simulink model "PID_houseROOMBA"  (R2024b)
settings: Solver=FixedStepAuto  StartTime=0.0  StopTime=inf  FixedStep=1/f_sim  RelTol=1e-3
model workspace (MATLAB code in the model file):
  | v_max=0.26;      % max |linear speed|
  | max_yaw=1.82;    % max |angular speed|
  | f_sim=1000;      % frequency
values from neighbouring files (symbols this model uses):
  crit_idces = -1    [Main_proj2_AstarROOMBA.m]
  path = path*res_BW-res_BW/2    [BW2GAZEBO.m]    (also in GAZEBO2BW.m = (path+res_BW/2)/res_BW; path_AstarFAST_1.mat = [-6.68726516648 -6.68556109776 -6.68385773308 -6.68215577647; path_AstarROOMBA_1.mat = [-6.7125 -6.6875 -6.6875 -6.6625 -6.6375 -6.6375 -6.6375 -6.; path_AstarROOMBA_2.mat = [4.8625 4.8375 4.8125 4.7875 4.7625 4.7375 4.7125 4.6875 4.6)
  reach_toll = 5*res    [Main_proj2_AstarFAST.m]    (also in Main_proj2_AstarROOMBA.m; Main_proj2_RRT.m = 70*mean(dist))
undefined symbols (not defined in the file or in its folder): Angular, DiscIntNeverNeededParam, Linear
libraries: robotlib x3, simulink x2, slpidlib x2
settings Model: Creator=eb  LastModifiedBy=vigno
settings OptimizationCC: DefaultParameterBehavior=Inlined  EnhancedBackFolding=on  PassReuseOutputArgsAs=Individual arguments  ZeroExternalMemoryAtStartup=off  ZeroInternalMemoryAtStartup=off  MaxStackSize=64  OptimizeBlockOrder=speed  DifferentSizesBufferReuse=on  OptimizationCustomize=off  EfficientTunableParamExpr=on
settings DebuggingCC: ParameterTunabilityLossMsg=error
settings HardwareCC: ProdBitPerPointer=32  ProdBitPerSizeT=32  ProdBitPerPtrDiffT=32  ProdLargestAtomicFloat=None  ProdIntDivRoundTo=Undefined  ProdEndianess=Unspecified  ProdWordSize=32  ProdHWDeviceType=Generic->Unspecified (assume 32-bit Generic)  UseEmbeddedCoderFeatures=off
settings SFSimCC: MATLABDynamicMemAlloc=off
settings RTWCC: Description=Embedded Coder  SystemTargetFile=ert.tlc  HardwareBoard=Robot Operating System (ROS)  TLCOptions="-aInlineSetEventsForThisBaseRateFcn=TLC_FALSE -aSuppressMultiTaskScheduler=TLC_FALSE  -aRateBasedStepFcn=0"  TemplateMakefile=ert_default_tmf  Toolchain=Catkin  TargetLang=C++
settings CodeAppCC: ForceParamTrailComments=on  IgnoreCustomStorageClasses=off  OperatorAnnotations=on  SimulinkDataObjDesc=on  SFDataObjDesc=on  InsertBlockDesc=on
settings ERTTargetCC: SupportNonInlinedSFcns=on

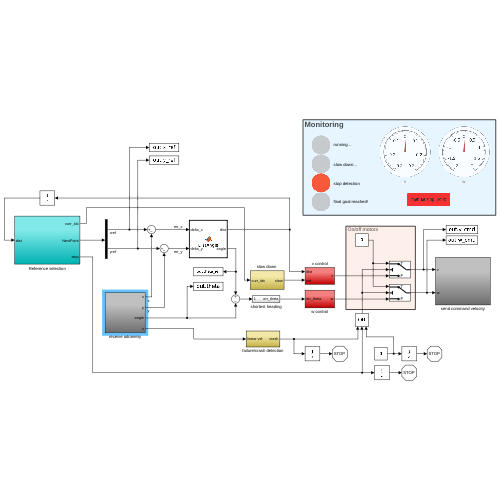
[thumbnail: Simulink's stored preview of the top-level diagram]
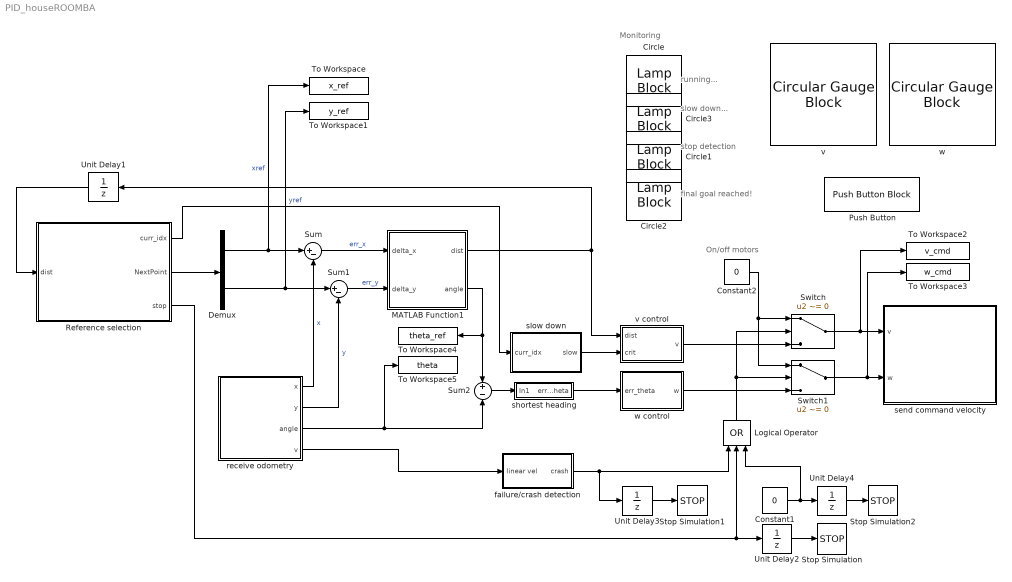
== system PID_houseROOMBA ==
  note: Monitoring
  note: running...
  note: On/off motors
  note: stop detection
  note: final goal reached!
  note: slow down...
  Circle{,1..3} (4 alike) : LampBlock  LabelPosition=Hide  Icon=Circle
  Constant1 : Constant  Value=0
  Constant2 : Constant  Value=0
  Demux : Demux  Outputs=2
  Logical Operator : Logic  Operator=OR  Inputs=3  AllPortsSameDT=off  OutDataTypeStr=boolean
  MATLAB Function1 : MATLAB Function  TreatAsAtomicUnit=on
  Push Button : PushButtonBlock  ButtonText=manual stop (hold)  OffValue=0.000000
  Reference selection : Subsystem
  Stop Simulation : Stop
  Stop Simulation1 : Stop
  Stop Simulation2 : Stop
  Sum : Sum  Inputs=|+-
  Sum1 : Sum  Inputs=|+-
  Sum2 : Sum  Inputs=+-
  Switch : Switch  Criteria=u2 ~= 0  SaturateOnIntegerOverflow=off  InputSameDT=off
  Switch1 : Switch  Criteria=u2 ~= 0  SaturateOnIntegerOverflow=off  InputSameDT=off
  To Workspace : ToWorkspace  VariableName=x_ref  SampleTime=-1
      settings: Save2DSignal=2-D array (concatenate along first dimension)
  To Workspace1 : ToWorkspace  VariableName=y_ref  SampleTime=-1
      settings: Save2DSignal=2-D array (concatenate along first dimension)
  To Workspace2 : ToWorkspace  VariableName=v_cmd  SampleTime=-1
      settings: Save2DSignal=2-D array (concatenate along first dimension)
  To Workspace3 : ToWorkspace  VariableName=w_cmd  SampleTime=-1
      settings: Save2DSignal=2-D array (concatenate along first dimension)
  To Workspace4 : ToWorkspace  VariableName=theta_ref  SampleTime=-1
      settings: Save2DSignal=2-D array (concatenate along first dimension)
  To Workspace5 : ToWorkspace  VariableName=theta  SampleTime=-1
      settings: Save2DSignal=2-D array (concatenate along first dimension)
  Unit Delay1 : UnitDelay  SampleTime=-1  HasFrameUpgradeWarning=on
  Unit Delay2 : UnitDelay  SampleTime=2  HasFrameUpgradeWarning=on
  Unit Delay3 : UnitDelay  SampleTime=0.5  HasFrameUpgradeWarning=on
  Unit Delay4 : UnitDelay  SampleTime=0.5  HasFrameUpgradeWarning=on
  failure/crash detection : Subsystem
  receive odometry : Subsystem
  send command velocity : Subsystem
  shortest heading : Subsystem
  "slow down " : Subsystem
  v : CircularGaugeBlock  LabelPosition=Hide  ScaleMin=-0.3  ScaleMax=0.3
  v control : Subsystem
  w : CircularGaugeBlock  LabelPosition=Hide  ScaleMin=-2  ScaleMax=2
  w control : Subsystem
  wires:
  Demux/1 -> Sum/1, To Workspace/1  "xref"
  Sum/1 -> MATLAB Function1/1(delta_x)  "err_x"
  Demux/2 -> Sum1/1, To Workspace1/1  "yref"
  Sum1/1 -> MATLAB Function1/2(delta_y)  "err_y"
  MATLAB Function1/2(angle) -> To Workspace4/1, Sum2/1
  MATLAB Function1/1(dist) -> v control/1(dist), Unit Delay1/1
  Sum2/1 -> shortest heading/1(In1)
  Unit Delay2/1 -> Stop Simulation/1
  Constant2/1 -> Switch1/1, Switch/1
  receive odometry/1(x) -> Sum/2  "x"
  receive odometry/2(y) -> Sum1/2  "y"
  receive odometry/3(angle) -> To Workspace5/1, Sum2/2
  Switch/1 -> To Workspace2/1, send command velocity/1(v)
  Switch1/1 -> To Workspace3/1, send command velocity/2(w)
  Reference selection/3(stop) -> Unit Delay2/1, Logical Operator/2
  Unit Delay1/1 -> Reference selection/1(dist)
  Reference selection/2(NextPoint) -> Demux/1
  receive odometry/4(v) -> failure/crash detection/1(linear vel)
  failure/crash detection/1(crash) -> Unit Delay3/1, Logical Operator/1
  Unit Delay3/1 -> Stop Simulation1/1
  Logical Operator/1 -> Switch1/2, Switch/2
  v control/1(v) -> Switch/3
  shortest heading/1(err_theta) -> w control/1(err_theta)
  "slow down "/1(slow) -> v control/2(crit)
  Reference selection/1(curr_idx) -> "slow down "/1(curr_idx)
  w control/1(w) -> Switch1/3
  Constant1/1 -> Logical Operator/3, Unit Delay4/1
  Unit Delay4/1 -> Stop Simulation2/1

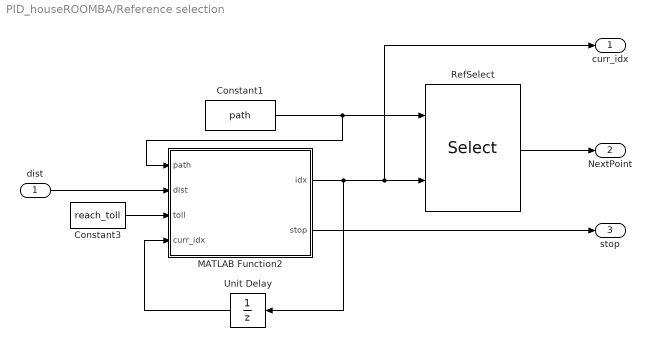
== system PID_houseROOMBA/Reference selection ==
  dist : Inport
  Constant1 : Constant  Value=path
  Constant3 : Constant  Value=reach_toll
  MATLAB Function2 : MATLAB Function  TreatAsAtomicUnit=on
  RefSelect : Selector  NumberOfDimensions=2  IndexOptions=Starting index (port),Select all  Indices=[1 3],[1:2]  OutputSizes=1,1
  Unit Delay : UnitDelay  SampleTime=-1  HasFrameUpgradeWarning=on
  curr_idx : Outport
  NextPoint : Outport  Port=2
  stop : Outport  Port=3
  wires:
  Constant3/1 -> MATLAB Function2/3(toll)
  dist/1 -> MATLAB Function2/2(dist)
  Unit Delay/1 -> MATLAB Function2/4(curr_idx)
  Constant1/1 -> MATLAB Function2/1(path), RefSelect/1
  RefSelect/1 -> NextPoint/1
  MATLAB Function2/2(stop) -> stop/1
  MATLAB Function2/1(idx) -> Unit Delay/1, curr_idx/1, RefSelect/2

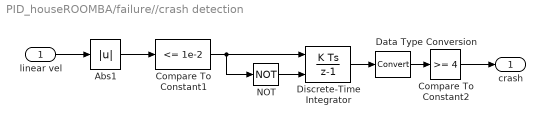
== system PID_houseROOMBA/failure//crash detection ==
  linear vel : Inport
  Abs1 : Abs  SaturateOnIntegerOverflow=off
  Compare To Constant1 : simulink/Logic and Bit Operations/Compare To Constant  relop=<=  const=1e-2  OutDataTypeStr=boolean
  Compare To Constant2 : simulink/Logic and Bit Operations/Compare To Constant  relop=>=  const=4  OutDataTypeStr=boolean
  Data Type Conversion : DataTypeConversion  SaturateOnIntegerOverflow=off  RndMeth=Floor
  Discrete-Time Integrator : DiscreteIntegrator  ExternalReset=rising  SampleTime=0.1  ICPrevOutput=DiscIntNeverNeededParam  ICPrevScaledInput=DiscIntNeverNeededParam
  NOT : Logic  Operator=NOT  IconShape=distinctive  AllPortsSameDT=off  OutDataTypeStr=boolean
  crash : Outport
  wires:
  linear vel/1 -> Abs1/1
  Abs1/1 -> Compare To Constant1/1
  Compare To Constant1/1 -> NOT/1, Discrete-Time Integrator/1
  Discrete-Time Integrator/1 -> Data Type Conversion/1
  NOT/1 -> Discrete-Time Integrator/2
  Compare To Constant2/1 -> crash/1
  Data Type Conversion/1 -> Compare To Constant2/1

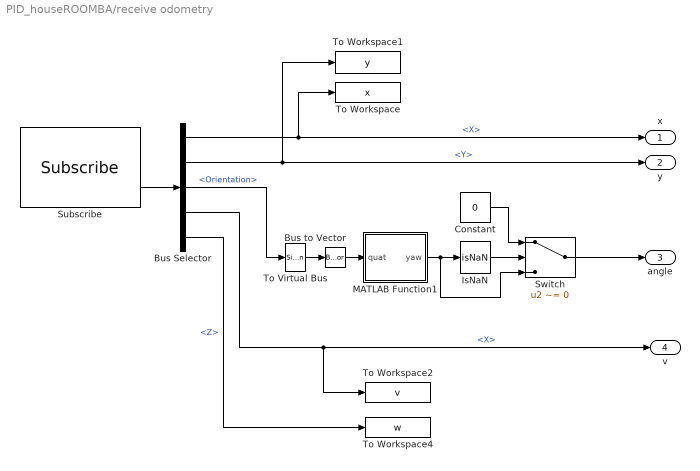
== system PID_houseROOMBA/receive odometry ==
  Bus Selector : BusSelector  OutputSignals=Pose.Pose.Position.X,Pose.Pose.Position.Y,Pose.Pose.Orientation,Twist.Twist.Linear.X,Twist.Twist.Angular.Z
  Bus to Vector : BusToVector
  Constant : Constant  Value=0
  IsNaN : RelationalOperator  Operator=isNaN  OutDataTypeStr=boolean  RndMeth=Simplest  InputSameDT=off
  MATLAB Function1 : MATLAB Function  TreatAsAtomicUnit=on
  Subscribe : robotlib/Subscribe  topicSource=Select from ROS network  topic=/odom  messageType=nav_msgs/Odometry  SampleTime=1/f_sim  legacyBusStruct=off  messageQueueLength=1
  Switch : Switch  Criteria=u2 ~= 0  SaturateOnIntegerOverflow=off  InputSameDT=off
  To Virtual Bus : SignalConversion  ConversionOutput=Virtual bus  OverrideOpt=off
  To Workspace : ToWorkspace  VariableName=x  SampleTime=-1
      settings: Save2DSignal=2-D array (concatenate along first dimension)
  To Workspace1 : ToWorkspace  VariableName=y  SampleTime=-1
      settings: Save2DSignal=2-D array (concatenate along first dimension)
  To Workspace2 : ToWorkspace  VariableName=v  SampleTime=-1
      settings: Save2DSignal=2-D array (concatenate along first dimension)
  To Workspace4 : ToWorkspace  VariableName=w  SampleTime=-1
      settings: Save2DSignal=2-D array (concatenate along first dimension)
  x : Outport
  y : Outport  Port=2
  angle : Outport  Port=3
  v : Outport  Port=4
  wires:
  Bus Selector/2 -> y/1, To Workspace1/1  "<Y>"
  Subscribe/2 -> Bus Selector/1
  Bus Selector/1 -> x/1, To Workspace/1  "<X>"
  Bus Selector/3 -> To Virtual Bus/1  "<Orientation>"
  Bus to Vector/1 -> MATLAB Function1/1(quat)
  To Virtual Bus/1 -> Bus to Vector/1
  MATLAB Function1/1(yaw) -> IsNaN/1, Switch/3
  IsNaN/1 -> Switch/2
  Constant/1 -> Switch/1
  Bus Selector/4 -> v/1, To Workspace2/1  "<X>"
  Bus Selector/5 -> To Workspace4/1  "<Z>"
  Switch/1 -> angle/1

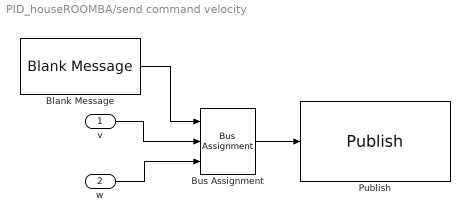
== system PID_houseROOMBA/send command velocity ==
  v : Inport
  w : Inport  Port=2
  Blank Message : robotlib/Blank Message  messageClass=Message  entityType=geometry_msgs/Twist  messageType=geometry_msgs/Twist  SampleTime=1/f_sim  legacyBusStruct=off
  Bus Assignment : BusAssignment  AssignedSignals=Linear.X,Angular.Z
  Publish : robotlib/Publish  topicSource=Select from ROS network  topic=/cmd_vel  messageType=geometry_msgs/Twist  legacyBusStruct=off  messageQueueLength=1
  wires:
  Blank Message/1 -> Bus Assignment/1
  v/1 -> Bus Assignment/2
  w/1 -> Bus Assignment/3
  Bus Assignment/1 -> Publish/1

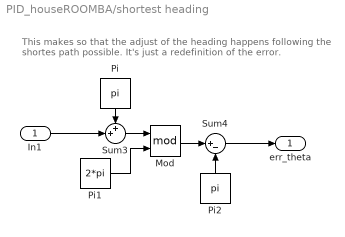
== system PID_houseROOMBA/shortest heading ==
  note: This makes so that the adjust of the heading happens following
      | the shortes path possible. It's just a redefinition of the error.
  In1 : Inport
  Mod : Math  Operator=mod
  Pi : Constant  Value=pi  OutDataTypeStr=Inherit: Inherit via back propagation
  Pi1 : Constant  Value=2*pi  OutDataTypeStr=Inherit: Inherit via back propagation
  Pi2 : Constant  Value=pi  OutDataTypeStr=Inherit: Inherit via back propagation
  Sum3 : Sum  Inputs=++|
  Sum4 : Sum  Inputs=|+-
  err_theta : Outport
  wires:
  Mod/1 -> Sum4/1
  Sum3/1 -> Mod/1
  Pi1/1 -> Mod/2
  Pi/1 -> Sum3/1
  Pi2/1 -> Sum4/2
  In1/1 -> Sum3/2
  Sum4/1 -> err_theta/1

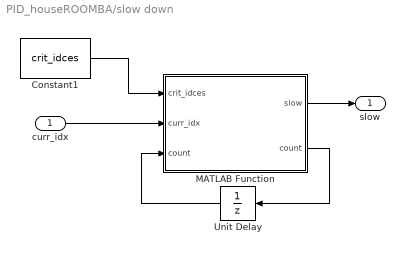
== system PID_houseROOMBA/slow down  ==
  curr_idx : Inport
  Constant1 : Constant  Value=crit_idces
  MATLAB Function : MATLAB Function  TreatAsAtomicUnit=on
  Unit Delay : UnitDelay  SampleTime=-1  HasFrameUpgradeWarning=on
  slow : Outport
  wires:
  Constant1/1 -> MATLAB Function/1(crit_idces)
  Unit Delay/1 -> MATLAB Function/3("count ")
  MATLAB Function/2(count) -> Unit Delay/1
  MATLAB Function/1(slow) -> slow/1
  curr_idx/1 -> MATLAB Function/2(curr_idx)

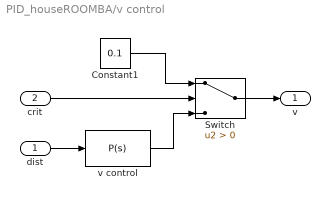
== system PID_houseROOMBA/v control ==
  dist : Inport
  crit : Inport  Port=2
  Constant1 : Constant  Value=0.1
  Switch : Switch  Criteria=u2 > Threshold  SaturateOnIntegerOverflow=off  InputSameDT=off
  v control : slpidlib/PID Controller  Controller=P  Form=Parallel  TimeDomain=Continuous-time  UseExternalTs=off  SampleTime=-1  IntegratorMethod=Forward Euler  FilterMethod=Forward Euler  ControllerParametersSource=internal  P=5  I=0.001  UseKiTs=off  D=1  UseExternalDerivativeSource=off  N=15  UseFilter=on  TunerSelectOption=Transfer Function Based (PID Tuner App)  InitialConditionSource=internal  InitialConditionForIntegrator=0  InitialConditionForFilter=0  DifferentiatorICPrevScaledInput=0  ExternalReset=none  TrackingMode=off  Kt=1  LimitOutput=on  SatLimitsSource=internal  UpperSaturationLimit=v_max  LowerSaturationLimit=-v_max  LinearizeAsGain=on  AntiWindupMode=clamping  Kb=1  LimitIntegrator=off  UpperIntegratorSaturationLimit=inf  LowerIntegratorSaturationLimit=-inf  POutMin=[]  POutMax=[]  IOutMin=[]  IOutMax=[]  DOutMin=[]  DOutMax=[]  NOutMin=[]  NOutMax=[]  SumOutMin=[]  SumOutMax=[]  SaturationOutMin=[]  SaturationOutMax=[]  PParamMin=[]  PParamMax=[]  IParamMin=[]  IParamMax=[]  DParamMin=[]  DParamMax=[]  NParamMin=[]  NParamMax=[]  KbParamMin=[]  KbParamMax=[]  KtParamMin=[]  KtParamMax=[]  KbOutMin=[]  KbOutMax=[]  KtOutMin=[]  KtOutMax=[]  IntegratorOutMin=[]  IntegratorOutMax=[]  FilterOutMin=[]  FilterOutMax=[]  SumI1OutMin=[]  SumI1OutMax=[]  SumI2OutMin=[]  SumI2OutMax=[]  SumI3OutMin=[]  SumI3OutMax=[]  SumI4OutMin=[]  SumI4OutMax=[]  SumDOutMin=[]  SumDOutMax=[]  DifferentiatorOutMin=[]  DifferentiatorOutMax=[]  FilterDiffOutCoefMin=[]  FilterDiffOutCoefMax=[]  ReciprocalOutMin=[]  ReciprocalOutMax=[]  SumDenOutMin=[]  SumDenOutMax=[]  SumNumOutMin=[]  SumNumOutMax=[]  DivideOutMin=[]  DivideOutMax=[]  UdiffTsProdOutMin=[]  UdiffTsProdOutMax=[]  NTsProdOutMin=[]  NTsProdOutMax=[]  UintegralTsProdOutMin=[]  UintegralTsProdOutMax=[]  UngainTsProdOutMin=[]  UngainTsProdOutMax=[]  ClampingZeroOutDataTypeStr=Inherit: Inherit via back propagation  ClampingZeroOutMin=[]  ClampingZeroOutMax=[]  FilterDenConstantOutDataTypeStr=Inherit: Inherit via back propagation  FilterDenConstantOutMin=[]  FilterDenConstantOutMax=[]  PCopyOutDataTypeStr=Inherit: Inherit via back propagation  PCopyOutMin=[]  PCopyOutMax=[]  NCopyOutDataTypeStr=Inherit: Inherit via back propagation  NCopyOutMin=[]  NCopyOutMax=[]  IntegratorContinuousStateAttributes=''  IntegratorStateMustResolveToSignalObject=off  IntegratorRTWStateStorageClass=Auto  FilterContinuousStateAttributes=''  FilterStateMustResolveToSignalObject=off  FilterRTWStateStorageClass=Auto  ParallelPVariant=InternalParameters  IdealPVariant=Disabled  IVariant=Disabled  DVariant=Disabled  IntegratorVariant=Disabled  SatVariant=Enabled  AWVariant=Disabled  PCopyVariant=Disabled  TRVariant=Disabled  FdbkBlocksVariant=Forward  IdealPFdbkVariant=Disabled  SatFdbkVariant=Disabled  DerivativeFilterVariant=Disabled  NVariant=Disabled  NCopyVariant=Disabled_SignalSpec  FilterICVariant=Disabled  IntegratorICVariant=Disabled  ExternalResetVariant=Disabled  TRSumVariant=Passthrough  SumFdbkVariant=Disabled  SumVariant=Passthrough_P  TsampFilterVariant=InternalTs  TsampNgainVariant=Passthrough  TsampIntegralVariant=Disabled_SignalSpec  ExternalSaturationOutDataTypeStr=Inherit: Same as second input  DerivativeSourceVariant=Disabled  PreIntVariant=InternalPreInt
  v : Outport
  wires:
  dist/1 -> v control/1
  Switch/1 -> v/1
  crit/1 -> Switch/2
  v control/1 -> Switch/3
  Constant1/1 -> Switch/1

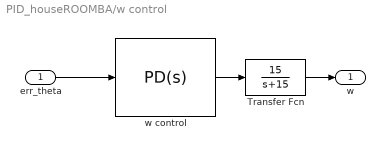
== system PID_houseROOMBA/w control ==
  err_theta : Inport
  Transfer Fcn : TransferFcn  Numerator=[15]  Denominator=[1 15]
  w control : slpidlib/PID Controller  Controller=PD  Form=Parallel  TimeDomain=Continuous-time  UseExternalTs=off  SampleTime=-1  IntegratorMethod=Forward Euler  FilterMethod=Forward Euler  ControllerParametersSource=internal  P=2.8  I=0.001  UseKiTs=off  D=1  UseExternalDerivativeSource=off  N=15  UseFilter=on  TunerSelectOption=Transfer Function Based (PID Tuner App)  InitialConditionSource=internal  InitialConditionForIntegrator=0  InitialConditionForFilter=0  DifferentiatorICPrevScaledInput=0  ExternalReset=none  TrackingMode=off  Kt=1  LimitOutput=on  SatLimitsSource=internal  UpperSaturationLimit=max_yaw  LowerSaturationLimit=-max_yaw  LinearizeAsGain=on  AntiWindupMode=clamping  Kb=1  LimitIntegrator=off  UpperIntegratorSaturationLimit=inf  LowerIntegratorSaturationLimit=-inf  POutMin=[]  POutMax=[]  IOutMin=[]  IOutMax=[]  DOutMin=[]  DOutMax=[]  NOutMin=[]  NOutMax=[]  SumOutMin=[]  SumOutMax=[]  SaturationOutMin=[]  SaturationOutMax=[]  PParamMin=[]  PParamMax=[]  IParamMin=[]  IParamMax=[]  DParamMin=[]  DParamMax=[]  NParamMin=[]  NParamMax=[]  KbParamMin=[]  KbParamMax=[]  KtParamMin=[]  KtParamMax=[]  KbOutMin=[]  KbOutMax=[]  KtOutMin=[]  KtOutMax=[]  IntegratorOutMin=[]  IntegratorOutMax=[]  FilterOutMin=[]  FilterOutMax=[]  SumI1OutMin=[]  SumI1OutMax=[]  SumI2OutMin=[]  SumI2OutMax=[]  SumI3OutMin=[]  SumI3OutMax=[]  SumI4OutMin=[]  SumI4OutMax=[]  SumDOutMin=[]  SumDOutMax=[]  DifferentiatorOutMin=[]  DifferentiatorOutMax=[]  FilterDiffOutCoefMin=[]  FilterDiffOutCoefMax=[]  ReciprocalOutMin=[]  ReciprocalOutMax=[]  SumDenOutMin=[]  SumDenOutMax=[]  SumNumOutMin=[]  SumNumOutMax=[]  DivideOutMin=[]  DivideOutMax=[]  UdiffTsProdOutMin=[]  UdiffTsProdOutMax=[]  NTsProdOutMin=[]  NTsProdOutMax=[]  UintegralTsProdOutMin=[]  UintegralTsProdOutMax=[]  UngainTsProdOutMin=[]  UngainTsProdOutMax=[]  ClampingZeroOutDataTypeStr=Inherit: Inherit via back propagation  ClampingZeroOutMin=[]  ClampingZeroOutMax=[]  FilterDenConstantOutDataTypeStr=Inherit: Inherit via back propagation  FilterDenConstantOutMin=[]  FilterDenConstantOutMax=[]  PCopyOutDataTypeStr=Inherit: Inherit via back propagation  PCopyOutMin=[]  PCopyOutMax=[]  NCopyOutDataTypeStr=Inherit: Inherit via back propagation  NCopyOutMin=[]  NCopyOutMax=[]  IntegratorContinuousStateAttributes=''  IntegratorStateMustResolveToSignalObject=off  IntegratorRTWStateStorageClass=Auto  FilterContinuousStateAttributes=''  FilterStateMustResolveToSignalObject=off  FilterRTWStateStorageClass=Auto  ParallelPVariant=InternalParameters  IdealPVariant=Disabled  IVariant=Disabled  DVariant=InternalParameters  IntegratorVariant=Disabled  SatVariant=Enabled  AWVariant=Disabled  PCopyVariant=Disabled  TRVariant=Disabled  FdbkBlocksVariant=Forward  IdealPFdbkVariant=Disabled  SatFdbkVariant=Disabled  DerivativeFilterVariant=ContFilter  NVariant=InternalParameters  NCopyVariant=Disabled  FilterICVariant=InternalICsFilter  IntegratorICVariant=Disabled  ExternalResetVariant=Disabled  TRSumVariant=Passthrough  SumFdbkVariant=Disabled  SumVariant=Sum_PD  TsampFilterVariant=InternalTs  TsampNgainVariant=Passthrough  TsampIntegralVariant=Disabled_SignalSpec  ExternalSaturationOutDataTypeStr=Inherit: Same as second input  DerivativeSourceVariant=ErrorSignal  PreIntVariant=InternalPreInt
  w : Outport
  wires:
  err_theta/1 -> w control/1
  w control/1 -> Transfer Fcn/1
  Transfer Fcn/1 -> w/1

== matlab function PID_houseROOMBA/MATLAB Function1 ==
  data: delta_x input; dist output; delta_y input; angle output
function [dist,angle]=DistAngle(delta_x,delta_y)

dist=sqrt(delta_x.^2+delta_y.^2);
angle=atan2(delta_y,delta_x);

end

== matlab function PID_houseROOMBA/slow down /MATLAB Function ==
  data: crit_idces input; slow output; curr_idx input; count input; count output
function [slow,count]=SlowDown(crit_idces,curr_idx,count)

if crit_idces==-1
    slow=false;
    count=-1;
else
    if count<=0
        count=1;
    elseif count>length(crit_idces)
        count=length(crit_idces);
    end
    
    if curr_idx>=crit_idces(count)-3 && curr_idx<crit_idces(count)+20
        slow=true;
    else
        slow=false;
    end
        
    if curr_idx==crit_idces(count)+20
        count=count+1;
    end
end

end

== matlab function PID_houseROOMBA/Reference selection/MATLAB Function2 ==
  data: path input; dist input; toll input; idx output; curr_idx input; stop output
function [idx,stop]=RefIdxSelect(path,dist,toll,curr_idx)

stop=false;
N_max=length(path);

if curr_idx<N_max && curr_idx>0
    if dist<toll
        idx=min(curr_idx+1,N_max);
    else
        idx=curr_idx;
    end
elseif curr_idx==0      % initial 'unit delay' condition
    idx=1;
else 
    idx=N_max;
    if dist<toll
        stop=true;
    end
end

end

== matlab function PID_houseROOMBA/receive odometry/MATLAB Function1 ==
  data: quat input; yaw output
function yaw=quat2yaw(quat)

q=zeros(1,4);

q(1)=quat(1);
q(2)=quat(2);
q(3)=quat(3);
q(4)=quat(4);

eul=quat2eul(q);

yaw=eul(3);

end
